simulink model "model_verification_discrete"  (R2024a)
settings: Solver=ode1  StartTime=0.0  StopTime=91  FixedStep=1/100  RelTol=1e-3
settings Model: Creator=ommore5807  LastModifiedBy=WickedSkyn
settings RTWCC: GPUComputeCapability=3.5

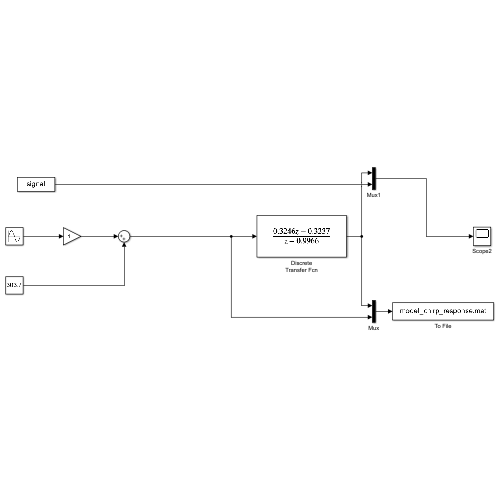
[thumbnail: Simulink's stored preview of the top-level diagram]
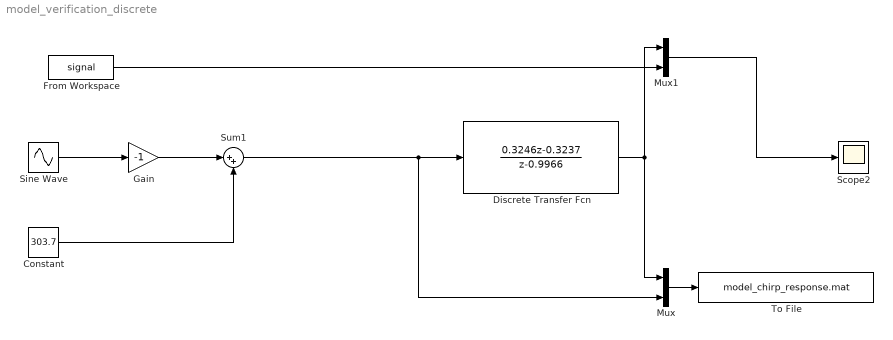
== system model_verification_discrete ==
  Constant : Constant  Value=303.7
  Discrete Transfer Fcn : DiscreteTransferFcn  Numerator=[0.3246, -0.3237]  Denominator=[ 1, -0.9966]
  From Workspace : FromWorkspace  VariableName=signal
  Gain : Gain  Gain=-1
  Mux : Mux  Inputs=2
  Mux1 : Mux  Inputs=2
  Scope2 : Scope
  Sine Wave : Sin  Amplitude=-279.06  Frequency=0.102  Phase=7.105  SampleTime=0
  Sum1 : Sum  Inputs=|++
  To File : ToFile  Filename=model_chirp_response.mat  MatrixName=model_step_response  SaveFormat=Timeseries
  wires:
  Discrete Transfer Fcn/1 -> Mux1/1, Mux/1
  Mux/1 -> To File/1
  Sum1/1 -> Mux/2, Discrete Transfer Fcn/1
  Sine Wave/1 -> Gain/1
  Gain/1 -> Sum1/1
  Constant/1 -> Sum1/2
  From Workspace/1 -> Mux1/2
  Mux1/1 -> Scope2/1
